simulink model "nms3D_2021"  (R2021a)
settings: Solver=ode15s  StartTime=0.0  StopTime=2  MaxStep=1e-2  RelTol=1e-2
StartFcn:
  | tic
StopFcn:
  | toc
  | 
  | 
  | %if GimbalLockFlag
  |  % fprintf(2, 'Almost reached Gimbal Lock of IMU. Simulation stopped.\n')
  | %end
  | 
  | %fprintf('Elapsed time: %4.2f sec (%4.2f%% realtime)\n', a, tout(end)/a*100)
values from neighbouring files (symbols this model uses):
  Balance02 = pMod(24:29)    [AssignSimulinkParams.m]    (also in assign_parameters.m = param(26:29))
  Balance13 = pMod(30:35)    [AssignSimulinkParams.m]    (also in assign_parameters.m = param(30:33))
  BalanceTrunk = pMod(22:23)    [AssignSimulinkParams.m]    (also in assign_parameters.m = param(22:23))
  BalanceTrunkLat = param(24:25)    [assign_parameters.m]
  BalanceTrunkLatOld = pMod(43:46)    [AssignSimulinkParams.m]    (also in assign_parameters.m = param(43:46))
  BalanceTrunkOld = param(49:53)    [assign_parameters.m]
  BasisStim = pMod(1:11)    [AssignSimulinkParams.m]    (also in assign_parameters.m = param(1:11))
  CompliantLeg = pMod(12:14)    [AssignSimulinkParams.m]    (also in assign_parameters.m = param(12:14))
  CompliantLegLat = pMod(15)    [AssignSimulinkParams.m]    (also in assign_parameters.m = param(15))
  PreventKneeOverextension = pMod(16:21)    [AssignSimulinkParams.m]    (also in assign_parameters.m = param(16:21))
  SwingCompLatOld = param(47:48)    [assign_parameters.m]
  Target02 = pMod(36:38)    [AssignSimulinkParams.m]    (also in assign_parameters.m = param(34:36))
  Target02_va = pMod(49:54)    [AssignSimulinkParams.m]    (also in assign_parameters.m = param(60:65))
  Target13 = pMod(39:41)    [AssignSimulinkParams.m]    (also in assign_parameters.m = param(37:39))
  Target13_va = pMod(55:60)    [AssignSimulinkParams.m]    (also in assign_parameters.m = param(66:71))
  theta0_world = param(59)    [assign_parameters.m]
  WramameiSL_1000 = readmatrix('WSL_1000_Norm_Sigmoid_MSE_cont.csv')    [nms3D_prep.m]
  ZramameiSL_1000 = readmatrix('ZSL_1000_Norm_Sigmoid_MSE_cont.csv')    [nms3D_prep.m]
undefined symbols (not defined in the file or in its folder): ICs, mParams, X, Y, Z
libraries: nesl_utility x106, sm_lib x87, simulink x70, eeGeneralControl x28, robotmaniplib x14, dspinverses x10, robotcorelib x5, dspmathops x3, vrlib x1, pid_lib x1
(part 6 of 8)

== system nms3D_2021/Supraspinal Level/Subsystem/Swing Leg Control ==
  note: Target Joint Angles
  note: Movement Plan
  note: These Time Delays (Low Pass Filters) have not been tested. If optimization causes problems, try to remove them or decrease delay value
  Left/Right : Inport
  Early/Late Swing : Inport  Port=2
  Compute Acceleration Profiles with Minimal Jerk Approach : Subsystem
  Compute Target States : Subsystem
  Inverse Dynamics: Left Leg : Subsystem
  Inverse Dynamics: Right Leg : Subsystem
  Mux : Mux
  NOT : Logic  Operator=NOT  AllPortsSameDT=off  OutDataTypeStr=boolean
  Terminator : Terminator
  To Workspace2 : ToWorkspace  VariableName=Acceleration  SampleTime=-1
      settings: Save2DSignal=2-D array (concatenate along first dimension)
  To Workspace3 : ToWorkspace  VariableName=TargetStates  SampleTime=-1
      settings: Save2DSignal=2-D array (concatenate along first dimension)
  long delay 1 : eeGeneralControl/Low-Pass Filter (Discrete or Continuous)  K=1  T=mParams.control.delays.long  B=inf  A=-inf  init_option=Inherited from block input  x0=0  Ts=-1
  long delay 2 : eeGeneralControl/Low-Pass Filter (Discrete or Continuous)  K=1  T=mParams.control.delays.long  B=inf  A=-inf  init_option=Inherited from block input  x0=0  Ts=-1
  Desired Torques Left Swing : Outport
  Desired Torques Right Swing : Outport  Port=2
  Interaction Wrench Right : Outport  Port=3
  Interaction Wrench Left : Outport  Port=4
  wires:
  Inverse Dynamics: Left Leg/2(Interaction Wrench) -> Interaction Wrench Right/1
  Compute Target States/3(Ankle Target) -> Mux/3, Compute Acceleration Profiles with Minimal Jerk Approach/3(Target State Ankle)
  Inverse Dynamics: Right Leg/2(Interaction Wrench) -> Interaction Wrench Left/1
  NOT/1 -> Inverse Dynamics: Left Leg/2(Enable)
  Compute Target States/2(Knee Target) -> Mux/2, Compute Acceleration Profiles with Minimal Jerk Approach/2(Target State Knee)
  Compute Target States/1(Hip Pitch Target) -> Mux/1, Compute Acceleration Profiles with Minimal Jerk Approach/1(Target State Hip Pitch)
  Inverse Dynamics: Right Leg/1(Desired Torques) -> long delay 2/1
  Mux/1 -> To Workspace3/1
  Compute Target States/4(Hip Roll Target) -> Mux/4, Compute Acceleration Profiles with Minimal Jerk Approach/4(Target State Hip Roll)
  Early/Late Swing/1 -> Compute Target States/2(Early/Late), Compute Acceleration Profiles with Minimal Jerk Approach/6(Early/Late Swing)
  Compute Acceleration Profiles with Minimal Jerk Approach/1("Desired Acceleration ") -> To Workspace2/1, Inverse Dynamics: Right Leg/1(Desired Acceleration), Inverse Dynamics: Left Leg/1(Desired Acceleration)
  Compute Acceleration Profiles with Minimal Jerk Approach/2(Joint Angles Swing) -> Terminator/1
  Inverse Dynamics: Left Leg/1(Desired Torques) -> long delay 1/1
  Left/Right/1 -> NOT/1, Inverse Dynamics: Right Leg/2(Enable), Compute Acceleration Profiles with Minimal Jerk Approach/5(Swing Right/Left), Compute Target States/1(Left/Right)
  long delay 1/1 -> Desired Torques Left Swing/1
  long delay 2/1 -> Desired Torques Right Swing/1

== system nms3D_2021/Body and Contact Model/L Leg/Foot/  XYZ Sensor Ball left1 ==
  note: Simplified IMU Model
  Frame Sensor : sm_lib/Frames and Transforms/Transform Sensor  MeasurementFrame=World  SenseAngle=off  SenseAxis=off  SenseAngle1=off  SenseAngle2=off  SenseAngle3=off  SenseQ=off  SenseR=on  SenseOmegaX=off  SenseOmegaY=off  SenseOmegaZ=off  SenseOmega1=off  SenseOmega2=off  SenseOmega3=off  SenseQDot=off  SenseRDot=off  SenseAlphaX=off  SenseAlphaY=off  SenseAlphaZ=off  SenseAlpha1=off  SenseAlpha2=off  SenseAlpha3=off  SenseQDDot=off  SenseRDDot=off  SenseX=on  SenseY=on  SenseZ=on  SenseRad=off  SenseAzim=off  SenseDist=off  SenseInc=off  SenseXDot=on  SenseYDot=on  SenseZDot=on  SenseRadDot=off  SenseAzimDot=off  SenseDistDot=off  SenseIncDot=off  SenseXDDot=off  SenseYDDot=off  SenseZDDot=off  SenseRadDDot=off  SenseAzimDDot=off  SenseDistDDot=off  SenseIncDDot=off
  Mux3 : Mux  Inputs=3
  Mux4 : Mux  Inputs=3
  PS-Simulink Converter : nesl_utility/PS-Simulink Converter  PhysicalDomain=network_engine_domain  SubClassName=ps_output  LeftPortType=input  RightPortType=output  PseudoPeriodic=off  Frequencies=[]  Unit=m  AffineConversion=off
      settings: SourceProductBaseCode=PW,SS
  PS-Simulink Converter1 : nesl_utility/PS-Simulink Converter  PhysicalDomain=network_engine_domain  SubClassName=ps_output  LeftPortType=input  RightPortType=output  PseudoPeriodic=off  Frequencies=[]  Unit=m  AffineConversion=off
      settings: SourceProductBaseCode=PW,SS
  PS-Simulink Converter2 : nesl_utility/PS-Simulink Converter  PhysicalDomain=network_engine_domain  SubClassName=ps_output  LeftPortType=input  RightPortType=output  PseudoPeriodic=off  Frequencies=[]  Unit=m/s  AffineConversion=off
      settings: SourceProductBaseCode=PW,SS
  PS-Simulink Converter3 : nesl_utility/PS-Simulink Converter  PhysicalDomain=network_engine_domain  SubClassName=ps_output  LeftPortType=input  RightPortType=output  PseudoPeriodic=off  Frequencies=[]  Unit=m/s  AffineConversion=off
      settings: SourceProductBaseCode=PW,SS
  PS-Simulink Converter4 : nesl_utility/PS-Simulink Converter  PhysicalDomain=network_engine_domain  SubClassName=ps_output  LeftPortType=input  RightPortType=output  PseudoPeriodic=off  Frequencies=[]  Unit=m  AffineConversion=off
      settings: SourceProductBaseCode=PW,SS
  PS-Simulink Converter5 : nesl_utility/PS-Simulink Converter  PhysicalDomain=network_engine_domain  SubClassName=ps_output  LeftPortType=input  RightPortType=output  PseudoPeriodic=off  Frequencies=[]  Unit=m/s  AffineConversion=off
      settings: SourceProductBaseCode=PW,SS
  PS-Simulink Converter6 : nesl_utility/PS-Simulink Converter  PhysicalDomain=network_engine_domain  SubClassName=ps_output  LeftPortType=input  RightPortType=output  PseudoPeriodic=off  Frequencies=[]  Unit=rad  AffineConversion=off
      settings: SourceProductBaseCode=PW,SS
  World Frame : sm_lib/Frames and Transforms/World Frame
  frame : PMIOPort  Side=Left
  p_bLH [m x3] : Outport  VectorParamsAs1DForOutWhenUnconnected=off
  v_bLH [m/s x3] : Outport  Port=2  VectorParamsAs1DForOutWhenUnconnected=off
  Rotation Matrix : Outport  Port=3  VectorParamsAs1DForOutWhenUnconnected=off
  wires:
  PS-Simulink Converter4/1 -> Mux3/3
  PS-Simulink Converter3/1 -> Mux4/2
  PS-Simulink Converter5/1 -> Mux4/3
  PS-Simulink Converter/1 -> Mux3/1
  Mux3/1 -> p_bLH [m x3]/1
  Mux4/1 -> v_bLH [m/s x3]/1
  PS-Simulink Converter2/1 -> Mux4/1
  PS-Simulink Converter1/1 -> Mux3/2
  PS-Simulink Converter6/1 -> Rotation Matrix/1
  connections:
  Frame Sensor/RConn1 -- frame/RConn1
  World Frame/RConn1 -- Frame Sensor/LConn1
  Frame Sensor/RConn3 -- PS-Simulink Converter/LConn1
  Frame Sensor/RConn4 -- PS-Simulink Converter1/LConn1
  Frame Sensor/RConn5 -- PS-Simulink Converter4/LConn1
  Frame Sensor/RConn6 -- PS-Simulink Converter2/LConn1
  Frame Sensor/RConn7 -- PS-Simulink Converter3/LConn1
  Frame Sensor/RConn8 -- PS-Simulink Converter5/LConn1
  Frame Sensor/RConn2 -- PS-Simulink Converter6/LConn1

== system nms3D_2021/Body and Contact Model/R Leg/Foot1/  XYZ Sensor  ==
  note: Simplified IMU Model
  Frame Sensor : sm_lib/Frames and Transforms/Transform Sensor  MeasurementFrame=World  SenseAngle=off  SenseAxis=off  SenseAngle1=off  SenseAngle2=off  SenseAngle3=off  SenseQ=off  SenseR=off  SenseOmegaX=off  SenseOmegaY=off  SenseOmegaZ=off  SenseOmega1=off  SenseOmega2=off  SenseOmega3=off  SenseQDot=off  SenseRDot=off  SenseAlphaX=off  SenseAlphaY=off  SenseAlphaZ=off  SenseAlpha1=off  SenseAlpha2=off  SenseAlpha3=off  SenseQDDot=off  SenseRDDot=off  SenseX=on  SenseY=on  SenseZ=on  SenseRad=off  SenseAzim=off  SenseDist=off  SenseInc=off  SenseXDot=on  SenseYDot=on  SenseZDot=on  SenseRadDot=off  SenseAzimDot=off  SenseDistDot=off  SenseIncDot=off  SenseXDDot=off  SenseYDDot=off  SenseZDDot=off  SenseRadDDot=off  SenseAzimDDot=off  SenseDistDDot=off  SenseIncDDot=off
  Mux3 : Mux  Inputs=3
  Mux4 : Mux  Inputs=3
  PS-Simulink Converter : nesl_utility/PS-Simulink Converter  PhysicalDomain=network_engine_domain  SubClassName=ps_output  LeftPortType=input  RightPortType=output  PseudoPeriodic=off  Frequencies=[]  Unit=m  AffineConversion=off
      settings: SourceProductBaseCode=PW,SS
  PS-Simulink Converter1 : nesl_utility/PS-Simulink Converter  PhysicalDomain=network_engine_domain  SubClassName=ps_output  LeftPortType=input  RightPortType=output  PseudoPeriodic=off  Frequencies=[]  Unit=m  AffineConversion=off
      settings: SourceProductBaseCode=PW,SS
  PS-Simulink Converter2 : nesl_utility/PS-Simulink Converter  PhysicalDomain=network_engine_domain  SubClassName=ps_output  LeftPortType=input  RightPortType=output  PseudoPeriodic=off  Frequencies=[]  Unit=m/s  AffineConversion=off
      settings: SourceProductBaseCode=PW,SS
  PS-Simulink Converter3 : nesl_utility/PS-Simulink Converter  PhysicalDomain=network_engine_domain  SubClassName=ps_output  LeftPortType=input  RightPortType=output  PseudoPeriodic=off  Frequencies=[]  Unit=m/s  AffineConversion=off
      settings: SourceProductBaseCode=PW,SS
  PS-Simulink Converter4 : nesl_utility/PS-Simulink Converter  PhysicalDomain=network_engine_domain  SubClassName=ps_output  LeftPortType=input  RightPortType=output  PseudoPeriodic=off  Frequencies=[]  Unit=m  AffineConversion=off
      settings: SourceProductBaseCode=PW,SS
  PS-Simulink Converter5 : nesl_utility/PS-Simulink Converter  PhysicalDomain=network_engine_domain  SubClassName=ps_output  LeftPortType=input  RightPortType=output  PseudoPeriodic=off  Frequencies=[]  Unit=m/s  AffineConversion=off
      settings: SourceProductBaseCode=PW,SS
  World Frame : sm_lib/Frames and Transforms/World Frame
  frame : PMIOPort  Side=Left
  p_bLH [m x3] : Outport  VectorParamsAs1DForOutWhenUnconnected=off
  v_bLH [m/s x3] : Outport  Port=2  VectorParamsAs1DForOutWhenUnconnected=off
  wires:
  PS-Simulink Converter4/1 -> Mux3/3
  PS-Simulink Converter3/1 -> Mux4/2
  PS-Simulink Converter5/1 -> Mux4/3
  PS-Simulink Converter/1 -> Mux3/1
  Mux3/1 -> p_bLH [m x3]/1
  Mux4/1 -> v_bLH [m/s x3]/1
  PS-Simulink Converter2/1 -> Mux4/1
  PS-Simulink Converter1/1 -> Mux3/2
  connections:
  Frame Sensor/RConn1 -- frame/RConn1
  World Frame/RConn1 -- Frame Sensor/LConn1
  Frame Sensor/RConn2 -- PS-Simulink Converter/LConn1
  Frame Sensor/RConn3 -- PS-Simulink Converter1/LConn1
  Frame Sensor/RConn4 -- PS-Simulink Converter4/LConn1
  Frame Sensor/RConn5 -- PS-Simulink Converter2/LConn1
  Frame Sensor/RConn6 -- PS-Simulink Converter3/LConn1
  Frame Sensor/RConn7 -- PS-Simulink Converter5/LConn1

== system nms3D_2021/Body and Contact Model/R Leg/Foot1/  XYZ Sensor Ball left1 ==
  note: Simplified IMU Model
  Frame Sensor : sm_lib/Frames and Transforms/Transform Sensor  MeasurementFrame=World  SenseAngle=off  SenseAxis=off  SenseAngle1=off  SenseAngle2=off  SenseAngle3=off  SenseQ=off  SenseR=on  SenseOmegaX=off  SenseOmegaY=off  SenseOmegaZ=off  SenseOmega1=off  SenseOmega2=off  SenseOmega3=off  SenseQDot=off  SenseRDot=off  SenseAlphaX=off  SenseAlphaY=off  SenseAlphaZ=off  SenseAlpha1=off  SenseAlpha2=off  SenseAlpha3=off  SenseQDDot=off  SenseRDDot=off  SenseX=on  SenseY=on  SenseZ=on  SenseRad=off  SenseAzim=off  SenseDist=off  SenseInc=off  SenseXDot=on  SenseYDot=on  SenseZDot=on  SenseRadDot=off  SenseAzimDot=off  SenseDistDot=off  SenseIncDot=off  SenseXDDot=off  SenseYDDot=off  SenseZDDot=off  SenseRadDDot=off  SenseAzimDDot=off  SenseDistDDot=off  SenseIncDDot=off
  Mux3 : Mux  Inputs=3
  Mux4 : Mux  Inputs=3
  PS-Simulink Converter : nesl_utility/PS-Simulink Converter  PhysicalDomain=network_engine_domain  SubClassName=ps_output  LeftPortType=input  RightPortType=output  PseudoPeriodic=off  Frequencies=[]  Unit=m  AffineConversion=off
      settings: SourceProductBaseCode=PW,SS
  PS-Simulink Converter1 : nesl_utility/PS-Simulink Converter  PhysicalDomain=network_engine_domain  SubClassName=ps_output  LeftPortType=input  RightPortType=output  PseudoPeriodic=off  Frequencies=[]  Unit=m  AffineConversion=off
      settings: SourceProductBaseCode=PW,SS
  PS-Simulink Converter2 : nesl_utility/PS-Simulink Converter  PhysicalDomain=network_engine_domain  SubClassName=ps_output  LeftPortType=input  RightPortType=output  PseudoPeriodic=off  Frequencies=[]  Unit=m/s  AffineConversion=off
      settings: SourceProductBaseCode=PW,SS
  PS-Simulink Converter3 : nesl_utility/PS-Simulink Converter  PhysicalDomain=network_engine_domain  SubClassName=ps_output  LeftPortType=input  RightPortType=output  PseudoPeriodic=off  Frequencies=[]  Unit=m/s  AffineConversion=off
      settings: SourceProductBaseCode=PW,SS
  PS-Simulink Converter4 : nesl_utility/PS-Simulink Converter  PhysicalDomain=network_engine_domain  SubClassName=ps_output  LeftPortType=input  RightPortType=output  PseudoPeriodic=off  Frequencies=[]  Unit=m  AffineConversion=off
      settings: SourceProductBaseCode=PW,SS
  PS-Simulink Converter5 : nesl_utility/PS-Simulink Converter  PhysicalDomain=network_engine_domain  SubClassName=ps_output  LeftPortType=input  RightPortType=output  PseudoPeriodic=off  Frequencies=[]  Unit=m/s  AffineConversion=off
      settings: SourceProductBaseCode=PW,SS
  PS-Simulink Converter6 : nesl_utility/PS-Simulink Converter  PhysicalDomain=network_engine_domain  SubClassName=ps_output  LeftPortType=input  RightPortType=output  PseudoPeriodic=off  Frequencies=[]  Unit=rad  AffineConversion=off
      settings: SourceProductBaseCode=PW,SS
  World Frame : sm_lib/Frames and Transforms/World Frame
  frame : PMIOPort  Side=Left
  p_bLH [m x3] : Outport  VectorParamsAs1DForOutWhenUnconnected=off
  v_bLH [m/s x3] : Outport  Port=2  VectorParamsAs1DForOutWhenUnconnected=off
  Rotation Matrix : Outport  Port=3  VectorParamsAs1DForOutWhenUnconnected=off
  wires:
  PS-Simulink Converter4/1 -> Mux3/3
  PS-Simulink Converter3/1 -> Mux4/2
  PS-Simulink Converter5/1 -> Mux4/3
  PS-Simulink Converter/1 -> Mux3/1
  Mux3/1 -> p_bLH [m x3]/1
  Mux4/1 -> v_bLH [m/s x3]/1
  PS-Simulink Converter2/1 -> Mux4/1
  PS-Simulink Converter1/1 -> Mux3/2
  PS-Simulink Converter6/1 -> Rotation Matrix/1
  connections:
  Frame Sensor/RConn1 -- frame/RConn1
  World Frame/RConn1 -- Frame Sensor/LConn1
  Frame Sensor/RConn3 -- PS-Simulink Converter/LConn1
  Frame Sensor/RConn4 -- PS-Simulink Converter1/LConn1
  Frame Sensor/RConn5 -- PS-Simulink Converter4/LConn1
  Frame Sensor/RConn6 -- PS-Simulink Converter2/LConn1
  Frame Sensor/RConn7 -- PS-Simulink Converter3/LConn1
  Frame Sensor/RConn8 -- PS-Simulink Converter5/LConn1
  Frame Sensor/RConn2 -- PS-Simulink Converter6/LConn1

== system nms3D_2021/Body and Contact Model/Vestibular System/Align Axis/Compute Lateral Rotation ==
  Hip Left : Inport
  Hip Right : Inport  Port=2
  Constant : Constant  Value=[0 0 1]
  Constant1 : Constant
  Constant2 : Constant  Value=-1
  Dot Product : DotProduct  InputSameDT=on  OutDataTypeStr=Inherit: Inherit via internal rule
  Minus : Sum  Inputs=+-
  Normalization : dspmathops/Normalization  NormType=2-norm  Bias=1e-10  NormOver=Each column  Dimension=1  roundingMode=Floor  overflowMode=off  accumDataTypeStr=Inherit: Same as product output  accumLastDataTypeStr=Inherit: Same as product output  outputDataTypeStr=Inherit: Same as product output  outputMin=[]  outputMax=[]  outputLastDataTypeStr=Inherit: Same as product output
  Product : Product
  Selector : Selector  InputPortWidth=3  IndexOptions=Index vector (dialog)  Indices=[2]  OutputSizes=1
  Switch : Switch  Criteria=u2 > Threshold
  Trigonometric Function : Trigonometry  Operator=acos
  Lateral Rotation : Outport
  wires:
  Hip Right/1 -> Minus/1
  Selector/1 -> Switch/2
  Product/1 -> Lateral Rotation/1
  Constant2/1 -> Switch/1
  Constant/1 -> Dot Product/1
  Constant1/1 -> Switch/3
  Switch/1 -> Product/1
  Trigonometric Function/1 -> Product/2
  Minus/1 -> Normalization/1
  Normalization/1 -> Dot Product/2, Selector/1
  Dot Product/1 -> Trigonometric Function/1
  Hip Left/1 -> Minus/2

== system nms3D_2021/Body and Contact Model/Vestibular System/Align Axis/Compute Saggital Rotation ==
  Hip Position Left [m] : Inport
  Hip Position Right [m] : Inport  Port=2
  Trunk Position [m] : Inport  Port=3
  Constant : Constant  Value=[0 1 0]
  Constant1 : Constant
  Constant2 : Constant  Value=-1
  Dot Product : DotProduct  InputSameDT=on  OutDataTypeStr=Inherit: Inherit via internal rule
  Gain : Gain  Gain=[0.5 0.5 0]
  Gain1 : Gain  Gain=[1 1 0]
  Minus : Sum
  Minus1 : Sum  Inputs=+-
  Normalization : dspmathops/Normalization  NormType=2-norm  Bias=1e-10  NormOver=Each column  Dimension=1  roundingMode=Floor  overflowMode=off  accumDataTypeStr=Inherit: Same as product output  accumLastDataTypeStr=Inherit: Same as product output  outputDataTypeStr=Inherit: Same as product output  outputMin=[]  outputMax=[]  outputLastDataTypeStr=Inherit: Same as product output
  Product : Product
  Selector : Selector  InputPortWidth=3  IndexOptions=Index vector (dialog)  Indices=[1]  OutputSizes=1
  Switch : Switch  Criteria=u2 > Threshold
  Trigonometric Function : Trigonometry  Operator=acos
  Saggital Rotation : Outport
  wires:
  Hip Position Right [m]/1 -> Minus/1
  Trigonometric Function/1 -> Product/2
  Constant/1 -> Dot Product/1
  Dot Product/1 -> Trigonometric Function/1
  Hip Position Left [m]/1 -> Minus/2
  Minus/1 -> Gain/1
  Gain/1 -> Minus1/2
  Trunk Position [m]/1 -> Gain1/1
  Minus1/1 -> Normalization/1
  Selector/1 -> Switch/2
  Constant1/1 -> Switch/3
  Constant2/1 -> Switch/1
  Switch/1 -> Product/1
  Product/1 -> Saggital Rotation/1
  Gain1/1 -> Minus1/1
  Normalization/1 -> Selector/1, Dot Product/2

== system nms3D_2021/Muscle Actuation Layer/Muscles Left/Muscle Dynamics (Vectorized)1/BE force-length relation ==
  note: Buffer Elasticity BE
  lce [lopt] : Inport
  Constant1 : Constant  Value=1-mParams.muscles.w
  Math Function : Math  Operator=square  SignedPower=on  SaturateOnIntegerOverflow=on
  Sum4 : Sum  Inputs=|+-  InputSameDT=on  SaturateOnIntegerOverflow=on  OutDataTypeStr=Inherit: Same as first input
  buffer engaged? : simulink/Logic and Bit Operations/Compare To Zero  relop=<  OutDataTypeStr=boolean  ZeroCross=off
  force of buffer elasticity : Product  Inputs=**
  reference strain [lslack] : Constant  Value=mParams.muscles.w/2
  relative strain : Product  Inputs=*/
  fbe [Fmax] : Outport  VectorParamsAs1DForOutWhenUnconnected=off
  wires:
  force of buffer elasticity/1 -> fbe [Fmax]/1
  Math Function/1 -> force of buffer elasticity/2
  buffer engaged?/1 -> force of buffer elasticity/1
  Constant1/1 -> Sum4/2
  Sum4/1 -> relative strain/1, buffer engaged?/1
  reference strain [lslack]/1 -> relative strain/2
  relative strain/1 -> Math Function/1
  lce [lopt]/1 -> Sum4/1

== system nms3D_2021/Muscle Actuation Layer/Muscles Left/Muscle Dynamics (Vectorized)1/CE force-length relation ==
  note: CE Force-Length Relationship
  lce [lopt] : Inport
  Abs : Abs
  Constant1 : Constant
  Constant2 : Constant  Value=3
  Gain : Gain  Gain=log(mParams.muscles.c)
  Math Function : Math  SignedPower=on  SaturateOnIntegerOverflow=on
  Math Function1 : Math  Operator=pow  SignedPower=on  SaturateOnIntegerOverflow=on
  Sum4 : Sum  Inputs=|+-  InputSameDT=on  SaturateOnIntegerOverflow=on  OutDataTypeStr=Inherit: Same as first input
  normalized position : Product  Inputs=*/
  relative width : Constant  Value=mParams.muscles.w
  fce [Fmax] : Outport  VectorParamsAs1DForOutWhenUnconnected=off
  wires:
  Math Function/1 -> fce [Fmax]/1
  Gain/1 -> Math Function/1
  Math Function1/1 -> Gain/1
  Constant2/1 -> Math Function1/2
  normalized position/1 -> Math Function1/1
  Abs/1 -> normalized position/1
  Sum4/1 -> Abs/1
  Constant1/1 -> Sum4/2
  relative width/1 -> normalized position/2
  lce [lopt]/1 -> Sum4/1

== system nms3D_2021/Muscle Actuation Layer/Muscles Left/Muscle Dynamics (Vectorized)1/CE inverse force-velocity relation ==
  note: CE Inverse Force-Velocity Relationship
  Fv[Fmax] : Inport
  1 : Product  Inputs=/*
  Constant{1,3..4,8} (4 alike) : Constant
  Constant2 : Constant  Value=mParams.muscles.N
  Curvature : Gain  Gain=mParams.muscles.K  SaturateOnIntegerOverflow=on  OutDataTypeStr=Inherit: Same as input  ParamDataTypeStr=Inherit: Same as input
  Curvature1 : Gain  Gain=7.56*mParams.muscles.K  SaturateOnIntegerOverflow=on  OutDataTypeStr=Inherit: Same as input  ParamDataTypeStr=Inherit: Same as input
  Logical Operator : Logic  Operator=NOT  AllPortsSameDT=off  OutDataTypeStr=boolean
  Logical Operator1 : Logic  Operator=NOT  AllPortsSameDT=off  OutDataTypeStr=boolean
  Slope : Gain  Gain=1e-2  SaturateOnIntegerOverflow=on  OutDataTypeStr=Inherit: Same as input  ParamDataTypeStr=Inherit: Same as input
  Sum1 : Sum  Inputs=|++  InputSameDT=on  SaturateOnIntegerOverflow=on  OutDataTypeStr=Inherit: Same as first input
  Sum2 : Sum  InputSameDT=on  SaturateOnIntegerOverflow=on  OutDataTypeStr=Inherit: Same as first input
  Sum3 : Sum  Inputs=++|  InputSameDT=on  SaturateOnIntegerOverflow=on  OutDataTypeStr=Inherit: Same as first input
  Sum4 : Sum  Inputs=|+-  InputSameDT=on  SaturateOnIntegerOverflow=on  OutDataTypeStr=Inherit: Same as first input
  Sum5 : Sum  Inputs=|-+  InputSameDT=on  SaturateOnIntegerOverflow=on  OutDataTypeStr=Inherit: Same as first input
  Sum6 : Sum  Inputs=-+|  InputSameDT=on  SaturateOnIntegerOverflow=on  OutDataTypeStr=Inherit: Same as first input
  Sum7 : Sum  Inputs=|++  InputSameDT=on  SaturateOnIntegerOverflow=on  OutDataTypeStr=Inherit: Same as first input
  Sum8 : Sum  Inputs=+-|  InputSameDT=on  SaturateOnIntegerOverflow=on  OutDataTypeStr=Inherit: Same as first input
  Sum9 : Sum  InputSameDT=on  SaturateOnIntegerOverflow=on  OutDataTypeStr=Inherit: Same as first input
  extension force within bound? : simulink/Logic and Bit Operations/Compare To Constant  relop=<=  const=mParams.muscles.N  OutDataTypeStr=boolean  ZeroCross=off
  force indicating contraction? : simulink/Logic and Bit Operations/Compare To Constant  relop=<=  const=1  OutDataTypeStr=boolean  ZeroCross=off
  v_concentric : Product  Inputs=*/
  v_concentric1 : Product  Inputs=**
  v_excentric <=N 1 : Product  Inputs=***
  v_excentric <N : Product  Inputs=*/
  v_excentric >N : Product  Inputs=**
  v[vmax] : Outport  VectorParamsAs1DForOutWhenUnconnected=off
  wires:
  Sum2/1 -> Sum9/2
  v_excentric <=N 1/1 -> Sum2/1
  Logical Operator1/1 -> v_excentric >N/1
  v_excentric >N/1 -> Sum2/2
  Logical Operator/1 -> v_excentric <=N 1/1
  Fv[Fmax]/1 -> extension force within bound?/1, force indicating contraction?/1, Curvature/1, Sum4/1, Sum6/2
  extension force within bound?/1 -> Logical Operator1/1, v_excentric <=N 1/3
  force indicating contraction?/1 -> Logical Operator/1, v_concentric1/2
  Sum1/1 -> v_excentric >N/2
  v_concentric1/1 -> Sum9/1
  v_excentric <N/1 -> v_excentric <=N 1/2
  Constant3/1 -> Sum5/1
  Sum5/1 -> 1/1
  Constant2/1 -> Sum5/2, Sum6/1
  Sum6/1 -> Slope/1, 1/2
  Constant8/1 -> Sum1/2
  Slope/1 -> Sum1/1
  Sum9/1 -> v[vmax]/1
  v_concentric/1 -> v_concentric1/1
  Sum7/1 -> v_excentric <N/1
  Sum8/1 -> v_excentric <N/2
  Curvature1/1 -> Sum8/2
  Constant4/1 -> Sum8/1, Sum7/2
  1/1 -> Curvature1/1, Sum7/1
  Sum3/1 -> v_concentric/2
  Sum4/1 -> v_concentric/1
  Constant1/1 -> Sum3/1, Sum4/2
  Curvature/1 -> Sum3/2

== system nms3D_2021/Muscle Actuation Layer/Muscles Left/Muscle Dynamics (Vectorized)1/PE force-length relation ==
  note: Parallel Elasticity PE
  lce [lopt] : Inport
  Constant3 : Constant
  Math Function2 : Math  Operator=square  SignedPower=on  SaturateOnIntegerOverflow=on
  Sum1 : Sum  Inputs=|+-  InputSameDT=on  SaturateOnIntegerOverflow=on  OutDataTypeStr=Inherit: Same as first input
  force of buffer elasticity : Product  Inputs=**
  parallel elasticity engaged? : simulink/Logic and Bit Operations/Compare To Zero  relop=>  OutDataTypeStr=boolean  ZeroCross=off
  reference strain [lopt] : Constant  Value=mParams.muscles.w
  relative strain : Product  Inputs=*/
  fpe [Fmax] : Outport  VectorParamsAs1DForOutWhenUnconnected=off
  wires:
  parallel elasticity engaged?/1 -> force of buffer elasticity/1
  force of buffer elasticity/1 -> fpe [Fmax]/1
  Math Function2/1 -> force of buffer elasticity/2
  relative strain/1 -> Math Function2/1
  reference strain [lopt]/1 -> relative strain/2
  Sum1/1 -> relative strain/1, parallel elasticity engaged?/1
  Constant3/1 -> Sum1/2
  lce [lopt]/1 -> Sum1/1

== system nms3D_2021/Muscle Actuation Layer/Muscles Left/Muscle Dynamics (Vectorized)1/SE force-length relation ==
  note: SE Force-Length Relationship
  lse [lslack] : Inport
  Constant1 : Constant
  Math Function : Math  Operator=square  SignedPower=on  SaturateOnIntegerOverflow=on
  Sum4 : Sum  Inputs=|+-  InputSameDT=on  SaturateOnIntegerOverflow=on  OutDataTypeStr=Inherit: Same as first input
  force above slack length : Product  Inputs=**
  greater than slack length? : simulink/Logic and Bit Operations/Compare To Zero  relop=>  OutDataTypeStr=boolean  ZeroCross=off
  reference strain [lslack] : Constant  Value=mParams.muscles.eref
  relative strain : Product  Inputs=*/
  fse [Fmax] : Outport  VectorParamsAs1DForOutWhenUnconnected=off
  wires:
  force above slack length/1 -> fse [Fmax]/1
  greater than slack length?/1 -> force above slack length/1
  Sum4/1 -> relative strain/1, greater than slack length?/1
  reference strain [lslack]/1 -> relative strain/2
  relative strain/1 -> Math Function/1
  lse [lslack]/1 -> Sum4/1
  Math Function/1 -> force above slack length/2
  Constant1/1 -> Sum4/2

== system nms3D_2021/Muscle Actuation Layer/Muscles Left/Muscle Torque Contributions1/Subsystem ==
  F VAS : Inport
  Moment Arm VAS : Inport  Port=2
  F SOL : Inport  Port=3
  Moment Arm SOL : Inport  Port=4
  Constant : Constant  Value=mParams.muscles.FmaxVec(7)
  Constant1 : Constant  Value=mParams.muscles.FmaxVec(10)
  Divide2 : Product  Inputs=*/
  Product{7..8,11..12} (4 alike) : Product
  Sum4 : Sum
  Sum6 : Sum
  "Leg Torque " : Outport
  wires:
  Sum4/1 -> Divide2/2
  Divide2/1 -> "Leg Torque "/1
  Moment Arm SOL/1 -> Product7/1, Product11/2
  Product11/1 -> Sum6/2
  Constant/1 -> Product8/2
  F VAS/1 -> Product12/1
  Moment Arm VAS/1 -> Product8/1, Product12/2
  Product7/1 -> Sum4/2
  F SOL/1 -> Product11/1
  Sum6/1 -> Divide2/1
  Product12/1 -> Sum6/1
  Constant1/1 -> Product7/2
  Product8/1 -> Sum4/1

== system nms3D_2021/Muscle Actuation Layer/Muscles Right/Muscle Dynamics (Vectorized)/BE force-length relation ==
  note: Buffer Elasticity BE
  lce [lopt] : Inport
  Constant1 : Constant  Value=1-mParams.muscles.w
  Math Function : Math  Operator=square  SignedPower=on  SaturateOnIntegerOverflow=on
  Sum4 : Sum  Inputs=|+-  InputSameDT=on  SaturateOnIntegerOverflow=on  OutDataTypeStr=Inherit: Same as first input
  buffer engaged? : simulink/Logic and Bit Operations/Compare To Zero  relop=<  OutDataTypeStr=boolean  ZeroCross=off
  force of buffer elasticity : Product  Inputs=**
  reference strain [lslack] : Constant  Value=mParams.muscles.w/2
  relative strain : Product  Inputs=*/
  fbe [Fmax] : Outport  VectorParamsAs1DForOutWhenUnconnected=off
  wires:
  force of buffer elasticity/1 -> fbe [Fmax]/1
  Math Function/1 -> force of buffer elasticity/2
  buffer engaged?/1 -> force of buffer elasticity/1
  Constant1/1 -> Sum4/2
  Sum4/1 -> relative strain/1, buffer engaged?/1
  reference strain [lslack]/1 -> relative strain/2
  relative strain/1 -> Math Function/1
  lce [lopt]/1 -> Sum4/1

== system nms3D_2021/Muscle Actuation Layer/Muscles Right/Muscle Dynamics (Vectorized)/CE force-length relation ==
  note: CE Force-Length Relationship
  lce [lopt] : Inport
  Abs : Abs
  Constant1 : Constant
  Constant2 : Constant  Value=3
  Gain : Gain  Gain=log(mParams.muscles.c)
  Math Function : Math  SignedPower=on  SaturateOnIntegerOverflow=on
  Math Function1 : Math  Operator=pow  SignedPower=on  SaturateOnIntegerOverflow=on
  Sum4 : Sum  Inputs=|+-  InputSameDT=on  SaturateOnIntegerOverflow=on  OutDataTypeStr=Inherit: Same as first input
  normalized position : Product  Inputs=*/
  relative width : Constant  Value=mParams.muscles.w
  fce [Fmax] : Outport  VectorParamsAs1DForOutWhenUnconnected=off
  wires:
  Math Function/1 -> fce [Fmax]/1
  Gain/1 -> Math Function/1
  Math Function1/1 -> Gain/1
  Constant2/1 -> Math Function1/2
  normalized position/1 -> Math Function1/1
  Abs/1 -> normalized position/1
  Sum4/1 -> Abs/1
  Constant1/1 -> Sum4/2
  relative width/1 -> normalized position/2
  lce [lopt]/1 -> Sum4/1

== system nms3D_2021/Muscle Actuation Layer/Muscles Right/Muscle Dynamics (Vectorized)/CE inverse force-velocity relation ==
  note: CE Inverse Force-Velocity Relationship
  Fv[Fmax] : Inport
  1 : Product  Inputs=/*
  Constant{1,3..4,8} (4 alike) : Constant
  Constant2 : Constant  Value=mParams.muscles.N
  Curvature : Gain  Gain=mParams.muscles.K  SaturateOnIntegerOverflow=on  OutDataTypeStr=Inherit: Same as input  ParamDataTypeStr=Inherit: Same as input
  Curvature1 : Gain  Gain=7.56*mParams.muscles.K  SaturateOnIntegerOverflow=on  OutDataTypeStr=Inherit: Same as input  ParamDataTypeStr=Inherit: Same as input
  Logical Operator : Logic  Operator=NOT  AllPortsSameDT=off  OutDataTypeStr=boolean
  Logical Operator1 : Logic  Operator=NOT  AllPortsSameDT=off  OutDataTypeStr=boolean
  Slope : Gain  Gain=1e-2  SaturateOnIntegerOverflow=on  OutDataTypeStr=Inherit: Same as input  ParamDataTypeStr=Inherit: Same as input
  Sum1 : Sum  Inputs=|++  InputSameDT=on  SaturateOnIntegerOverflow=on  OutDataTypeStr=Inherit: Same as first input
  Sum2 : Sum  InputSameDT=on  SaturateOnIntegerOverflow=on  OutDataTypeStr=Inherit: Same as first input
  Sum3 : Sum  Inputs=++|  InputSameDT=on  SaturateOnIntegerOverflow=on  OutDataTypeStr=Inherit: Same as first input
  Sum4 : Sum  Inputs=|+-  InputSameDT=on  SaturateOnIntegerOverflow=on  OutDataTypeStr=Inherit: Same as first input
  Sum5 : Sum  Inputs=|-+  InputSameDT=on  SaturateOnIntegerOverflow=on  OutDataTypeStr=Inherit: Same as first input
  Sum6 : Sum  Inputs=-+|  InputSameDT=on  SaturateOnIntegerOverflow=on  OutDataTypeStr=Inherit: Same as first input
  Sum7 : Sum  Inputs=|++  InputSameDT=on  SaturateOnIntegerOverflow=on  OutDataTypeStr=Inherit: Same as first input
  Sum8 : Sum  Inputs=+-|  InputSameDT=on  SaturateOnIntegerOverflow=on  OutDataTypeStr=Inherit: Same as first input
  Sum9 : Sum  InputSameDT=on  SaturateOnIntegerOverflow=on  OutDataTypeStr=Inherit: Same as first input
  extension force within bound? : simulink/Logic and Bit Operations/Compare To Constant  relop=<=  const=mParams.muscles.N  OutDataTypeStr=boolean  ZeroCross=off
  force indicating contraction? : simulink/Logic and Bit Operations/Compare To Constant  relop=<=  const=1  OutDataTypeStr=boolean  ZeroCross=off
  v_concentric : Product  Inputs=*/
  v_concentric1 : Product  Inputs=**
  v_excentric <=N 1 : Product  Inputs=***
  v_excentric <N : Product  Inputs=*/
  v_excentric >N : Product  Inputs=**
  v[vmax] : Outport  VectorParamsAs1DForOutWhenUnconnected=off
  wires:
  Sum2/1 -> Sum9/2
  v_excentric <=N 1/1 -> Sum2/1
  Logical Operator1/1 -> v_excentric >N/1
  v_excentric >N/1 -> Sum2/2
  Logical Operator/1 -> v_excentric <=N 1/1
  Fv[Fmax]/1 -> extension force within bound?/1, force indicating contraction?/1, Curvature/1, Sum4/1, Sum6/2
  extension force within bound?/1 -> Logical Operator1/1, v_excentric <=N 1/3
  force indicating contraction?/1 -> Logical Operator/1, v_concentric1/2
  Sum1/1 -> v_excentric >N/2
  v_concentric1/1 -> Sum9/1
  v_excentric <N/1 -> v_excentric <=N 1/2
  Constant3/1 -> Sum5/1
  Sum5/1 -> 1/1
  Constant2/1 -> Sum5/2, Sum6/1
  Sum6/1 -> Slope/1, 1/2
  Constant8/1 -> Sum1/2
  Slope/1 -> Sum1/1
  Sum9/1 -> v[vmax]/1
  v_concentric/1 -> v_concentric1/1
  Sum7/1 -> v_excentric <N/1
  Sum8/1 -> v_excentric <N/2
  Curvature1/1 -> Sum8/2
  Constant4/1 -> Sum8/1, Sum7/2
  1/1 -> Curvature1/1, Sum7/1
  Sum3/1 -> v_concentric/2
  Sum4/1 -> v_concentric/1
  Constant1/1 -> Sum3/1, Sum4/2
  Curvature/1 -> Sum3/2

== system nms3D_2021/Muscle Actuation Layer/Muscles Right/Muscle Dynamics (Vectorized)/PE force-length relation ==
  note: Parallel Elasticity PE
  lce [lopt] : Inport
  Constant3 : Constant
  Math Function2 : Math  Operator=square  SignedPower=on  SaturateOnIntegerOverflow=on
  Sum1 : Sum  Inputs=|+-  InputSameDT=on  SaturateOnIntegerOverflow=on  OutDataTypeStr=Inherit: Same as first input
  force of buffer elasticity : Product  Inputs=**
  parallel elasticity engaged? : simulink/Logic and Bit Operations/Compare To Zero  relop=>  OutDataTypeStr=boolean  ZeroCross=off
  reference strain [lopt] : Constant  Value=mParams.muscles.w
  relative strain : Product  Inputs=*/
  fpe [Fmax] : Outport  VectorParamsAs1DForOutWhenUnconnected=off
  wires:
  parallel elasticity engaged?/1 -> force of buffer elasticity/1
  force of buffer elasticity/1 -> fpe [Fmax]/1
  Math Function2/1 -> force of buffer elasticity/2
  relative strain/1 -> Math Function2/1
  reference strain [lopt]/1 -> relative strain/2
  Sum1/1 -> relative strain/1, parallel elasticity engaged?/1
  Constant3/1 -> Sum1/2
  lce [lopt]/1 -> Sum1/1

== system nms3D_2021/Muscle Actuation Layer/Muscles Right/Muscle Dynamics (Vectorized)/SE force-length relation ==
  note: SE Force-Length Relationship
  lse [lslack] : Inport
  Constant1 : Constant
  Math Function : Math  Operator=square  SignedPower=on  SaturateOnIntegerOverflow=on
  Sum4 : Sum  Inputs=|+-  InputSameDT=on  SaturateOnIntegerOverflow=on  OutDataTypeStr=Inherit: Same as first input
  force above slack length : Product  Inputs=**
  greater than slack length? : simulink/Logic and Bit Operations/Compare To Zero  relop=>  OutDataTypeStr=boolean  ZeroCross=off
  reference strain [lslack] : Constant  Value=mParams.muscles.eref
  relative strain : Product  Inputs=*/
  fse [Fmax] : Outport  VectorParamsAs1DForOutWhenUnconnected=off
  wires:
  force above slack length/1 -> fse [Fmax]/1
  greater than slack length?/1 -> force above slack length/1
  Constant1/1 -> Sum4/2
  Sum4/1 -> relative strain/1, greater than slack length?/1
  relative strain/1 -> Math Function/1
  lse [lslack]/1 -> Sum4/1
  Math Function/1 -> force above slack length/2
  reference strain [lslack]/1 -> relative strain/2

== system nms3D_2021/Muscle Actuation Layer/Muscles Right/Muscle Torque Contributions/Subsystem ==
  F VAS : Inport
  Moment Arm VAS : Inport  Port=2
  F SOL : Inport  Port=3
  Moment Arm SOL : Inport  Port=4
  Constant : Constant  Value=mParams.muscles.FmaxVec(7)
  Constant1 : Constant  Value=mParams.muscles.FmaxVec(10)
  Divide2 : Product  Inputs=*/
  Product{7..8,11..12} (4 alike) : Product
  Sum4 : Sum
  Sum6 : Sum
  "Leg Torque " : Outport
  wires:
  Sum4/1 -> Divide2/2
  Divide2/1 -> "Leg Torque "/1
  Moment Arm SOL/1 -> Product7/1, Product11/2
  Product11/1 -> Sum6/2
  Constant/1 -> Product8/2
  F VAS/1 -> Product12/1
  Moment Arm VAS/1 -> Product8/1, Product12/2
  Product7/1 -> Sum4/2
  F SOL/1 -> Product11/1
  Sum6/1 -> Divide2/1
  Product12/1 -> Sum6/1
  Constant1/1 -> Product7/2
  Product8/1 -> Sum4/1

== system nms3D_2021/Supraspinal Level/Subsystem/Compute positives forces that generate desired torque profiles1/Left ==
  Desired Torques : Inport
  Angles : Inport  Port=2
  Constant : Constant  Value=WramameiSL_1000  VectorParams1D=off  SampleTime=-1
  Constant1 : Constant  Value=|
      | [1.666708374023437500e+01
      | -3.333266830444335938e+01]
  Constant2 : Constant  Value=ZramameiSL_1000
  Constant3 : Constant  Value=[-1/mParams.muscles.INV.r0 1/mParams.muscles.EVE.r0]
  Denorm : Gain  Gain=[2000, 1500, 3000, 1200, 6000, 350, 1500, 4000, 800]
  Matrix Concatenate : Concatenate  Mode=Multidimensional array
  Matrix Concatenate4 : Concatenate  NumInputs=3  Mode=Multidimensional array  ConcatenateDimension=2
  Matrix Multiply{1..3,8} (4 alike) : Product  Multiplication=Matrix(*)
  Multiply : Gain  Gain=1/960
  Multiply2 : Gain  Gain=1/3.0543
  Saturation : Saturate  UpperLimit=inf  LowerLimit=0  ZeroCross=off
  Saturation1 : Saturate  UpperLimit=inf  LowerLimit=0  ZeroCross=off
  Saturation2 : Saturate  UpperLimit=inf  LowerLimit=0  ZeroCross=off
  Selector : Selector  InputPortWidth=5  IndexOptions=Index vector (dialog)  Indices=[1 3 5]  OutputSizes=1
  Selector1 : Selector  InputPortWidth=5  IndexOptions=Index vector (dialog)  Indices=[3 5]  OutputSizes=1
  Selector2 : Selector  InputPortWidth=5  IndexOptions=Index vector (dialog)  Indices=4  OutputSizes=1
  Selector8 : Selector  InputPortWidth=5  IndexOptions=Index vector (dialog)  Indices=2  OutputSizes=1
  Transpose1 : Math  Operator=transpose  SaturateOnIntegerOverflow=on
  Transpose3 : Math  Operator=transpose  SaturateOnIntegerOverflow=on
  Transpose9 : Math  Operator=transpose  SaturateOnIntegerOverflow=on
  sigmoid : Subsystem
  Forces : Outport
  wires:
  Desired Torques/1 -> Selector/1, Selector2/1, Selector8/1
  Selector1/1 -> Multiply2/1
  Matrix Multiply2/1 -> Saturation/1
  Selector/1 -> Multiply/1
  Constant/1 -> Matrix Multiply3/2
  Constant2/1 -> Matrix Multiply2/2
  Angles/1 -> Selector1/1
  Matrix Multiply8/1 -> Saturation2/1
  Constant1/1 -> Transpose9/1
  Selector8/1 -> Matrix Multiply8/1
  Transpose9/1 -> Matrix Multiply8/2
  Saturation/1 -> Denorm/1
  Matrix Concatenate4/1 -> Forces/1
  Saturation2/1 -> Matrix Concatenate4/1
  Transpose3/1 -> Matrix Multiply3/1
  Matrix Concatenate/1 -> Transpose3/1  "tr"
  Denorm/1 -> Matrix Concatenate4/2
  Multiply/1 -> Matrix Concatenate/1
  Multiply2/1 -> Matrix Concatenate/2
  sigmoid/1(Out1) -> Matrix Multiply2/1
  Matrix Multiply3/1 -> sigmoid/1(In1)
  Selector2/1 -> Matrix Multiply1/1
  Transpose1/1 -> Matrix Multiply1/2
  Constant3/1 -> Transpose1/1
  Matrix Multiply1/1 -> Saturation1/1
  Saturation1/1 -> Matrix Concatenate4/3

== system nms3D_2021/Supraspinal Level/Subsystem/Compute positives forces that generate desired torque profiles1/Right ==
  Desired Torques : Inport
  Angles : Inport  Port=2
  Constant : Constant  Value=WramameiSL_1000  VectorParams1D=off  SampleTime=-1
  Constant1 : Constant  Value=|
      | [1.666708374023437500e+01
      | -3.333266830444335938e+01]
  Constant2 : Constant  Value=ZramameiSL_1000
  Constant3 : Constant  Value=[-1/mParams.muscles.INV.r0 1/mParams.muscles.EVE.r0]
  Denorm : Gain  Gain=[2000, 1500, 3000, 1200, 6000, 350, 1500, 4000, 800]
  Matrix Concatenate : Concatenate  Mode=Multidimensional array
  Matrix Concatenate4 : Concatenate  NumInputs=3  Mode=Multidimensional array  ConcatenateDimension=2
  Matrix Multiply{1..3,8} (4 alike) : Product  Multiplication=Matrix(*)
  Multiply : Gain  Gain=1/960
  Multiply2 : Gain  Gain=1/3.0543
  Saturation : Saturate  UpperLimit=inf  LowerLimit=0  ZeroCross=off
  Saturation1 : Saturate  UpperLimit=inf  LowerLimit=0  ZeroCross=off
  Saturation2 : Saturate  UpperLimit=inf  LowerLimit=0  ZeroCross=off
  Selector : Selector  InputPortWidth=5  IndexOptions=Index vector (dialog)  Indices=[1 3 5]  OutputSizes=1
  Selector1 : Selector  InputPortWidth=5  IndexOptions=Index vector (dialog)  Indices=[3 5]  OutputSizes=1
  Selector2 : Selector  InputPortWidth=5  IndexOptions=Index vector (dialog)  Indices=4  OutputSizes=1
  Selector8 : Selector  InputPortWidth=5  IndexOptions=Index vector (dialog)  Indices=2  OutputSizes=1
  Transpose1 : Math  Operator=transpose  SaturateOnIntegerOverflow=on
  Transpose3 : Math  Operator=transpose  SaturateOnIntegerOverflow=on
  Transpose9 : Math  Operator=transpose  SaturateOnIntegerOverflow=on
  sigmoid : Subsystem
  Forces : Outport
  wires:
  Desired Torques/1 -> Selector/1, Selector2/1, Selector8/1
  Selector1/1 -> Multiply2/1
  Matrix Multiply2/1 -> Saturation/1
  Selector/1 -> Multiply/1
  Constant/1 -> Matrix Multiply3/2
  Constant2/1 -> Matrix Multiply2/2
  Angles/1 -> Selector1/1
  Matrix Multiply8/1 -> Saturation2/1
  Constant1/1 -> Transpose9/1
  Selector8/1 -> Matrix Multiply8/1
  Transpose9/1 -> Matrix Multiply8/2
  Saturation/1 -> Denorm/1
  Matrix Concatenate4/1 -> Forces/1
  Saturation2/1 -> Matrix Concatenate4/1
  Transpose3/1 -> Matrix Multiply3/1
  Matrix Concatenate/1 -> Transpose3/1  "tr"
  Denorm/1 -> Matrix Concatenate4/2
  Multiply/1 -> Matrix Concatenate/1
  Multiply2/1 -> Matrix Concatenate/2
  sigmoid/1(Out1) -> Matrix Multiply2/1
  Matrix Multiply3/1 -> sigmoid/1(In1)
  Saturation1/1 -> Matrix Concatenate4/3
  Constant3/1 -> Transpose1/1
  Selector2/1 -> Matrix Multiply1/1
  Transpose1/1 -> Matrix Multiply1/2
  Matrix Multiply1/1 -> Saturation1/1

== system nms3D_2021/Supraspinal Level/Subsystem/Stance Leg Control/Balance Control Equation [Ankle Strategy] ==
  Add : Sum  Commented=on  Inputs=+--++
  Constant : Constant  Commented=on  Value=ICs.trunk.vx0
  Constant1 : Constant  Value=0.02
  From1 : From  Commented=on  GotoTag=m3  TagVisibility=global
  From2 : From  Commented=on  GotoTag=m0  TagVisibility=global
  From3 : From  Commented=on  GotoTag=m1  TagVisibility=global
  From4 : From  Commented=on  GotoTag=d  TagVisibility=global
  From5 : From  Commented=on  GotoTag=CoM_Velocity_rot  TagVisibility=global
  From6 : From  Commented=on  GotoTag=m2  TagVisibility=global
  From7 : From  Commented=on  GotoTag=v_mid  TagVisibility=global
  From8 : From  Commented=on  GotoTag=m4  TagVisibility=global
  Minus : Sum  Commented=on  Inputs=+-
  Product{1..4} (4 alike) : Product  Commented=on
  Scope : Scope  Commented=on
  Scope1 : Scope
  Selector6 : Selector  Commented=on  InputPortWidth=3  IndexOptions=Index vector (dialog)  Indices=[1]  OutputSizes=1
  To Workspace2 : ToWorkspace  Commented=on  VariableName=EndVelocity  SampleTime=-1
      settings: MaxDataPoints=1  Save2DSignal=2-D array (concatenate along first dimension)
  mean (1s) : Subsystem  Commented=on
  Desired Acceleration (CoM) : Outport
  wires:
  From5/1 -> Selector6/1
  Selector6/1 -> Product3/1
  From2/1 -> Add/1
  Product2/1 -> Add/2
  From4/1 -> Product2/2
  From3/1 -> Product2/1
  Product3/1 -> Add/3
  From6/1 -> Product3/2
  From7/1 -> mean (1s)/1(u), To Workspace2/1, Minus/2
  Minus/1 -> Product1/1
  From1/1 -> Product1/2
  Product1/1 -> Add/4
  Constant/1 -> Minus/1, Product4/1
  From8/1 -> Product4/2
  Product4/1 -> Add/5
  Constant1/1 -> Desired Acceleration (CoM)/1

== system nms3D_2021/Supraspinal Level/Subsystem/Stance Leg Control/Coordiante Transform Interaction Wrenches ==
  note: Transform sensory data into coordinates of the swing leg RBT model
  note: Transform wrench from world coordinates into world coordinates aligned with the walking direction of the model
  InteractionWrenchLeft : Inport
  InteractionWrenchRight : Inport  Port=2
  Left/Right : Inport  Port=3
  Create Adjoint : Subsystem
  Matrix Multiply1 : Product  Multiplication=Matrix(*)
  Mux1 : Mux  Inputs=2
  Switch : Switch  Criteria=u2 > Threshold  ZeroCross=off
  Switch1 : Switch  Criteria=u2 > Threshold  ZeroCross=off
  "Transform  Velocity from world to body " : Subsystem
  Transpose1 : Math  Operator=transpose  SaturateOnIntegerOverflow=on
  transform wrench from body to world frame1 : Subsystem
  Interaction Wrench [Hip Coordinates] : Outport
  tag scope: RotationalVelocityTrunk=global, TranslationalVelocityTrunk=global
  wires:
  Left/Right/1 -> Switch1/2, Switch/2
  InteractionWrenchLeft/1 -> Switch/1
  [RotationTrunk] -> transform wrench from body to world frame1/2(CoM Rot)
  Mux1/1 -> Matrix Multiply1/2
  Switch1/1 -> Create Adjoint/1(R)
  [CoM_Position] -> transform wrench from body to world frame1/1("CoM Pos ")
  "Transform  Velocity from world to body "/1(Translational Velocity [body]) -> [TranslationalVelocityTrunk]
  transform wrench from body to world frame1/2(torque) -> Mux1/1
  transform wrench from body to world frame1/1(body-world jacobian) -> "Transform  Velocity from world to body "/1(body-world jacobian)
  transform wrench from body to world frame1/3(force) -> Mux1/2
  [RotationVelocityTrunk] -> "Transform  Velocity from world to body "/3(rotational velocity [world])
  Create Adjoint/1(Ad(R)) -> Transpose1/1
  "Transform  Velocity from world to body "/2(Rotational Velocity [body]) -> [RotationalVelocityTrunk]
  [CoM_Velocity] -> "Transform  Velocity from world to body "/2(translational velocity [world])
  Transpose1/1 -> Matrix Multiply1/1
  Switch/1 -> transform wrench from body to world frame1/3(wrench [rbt model])
  [RotationMatrixRightFoot] -> Switch1/3
  [RotationMatrixLeftFoot] -> Switch1/1
  InteractionWrenchRight/1 -> Switch/3
  Matrix Multiply1/1 -> Interaction Wrench [Hip Coordinates]/1
